simulink model "laba4"  (R2016b)
settings: Solver=VariableStepAuto  StartTime=0.0  StopTime=0.35  MaxStep=0.001  RelTol=1e-3
settings Model: Creator=Admin  LastModifiedBy=Admin

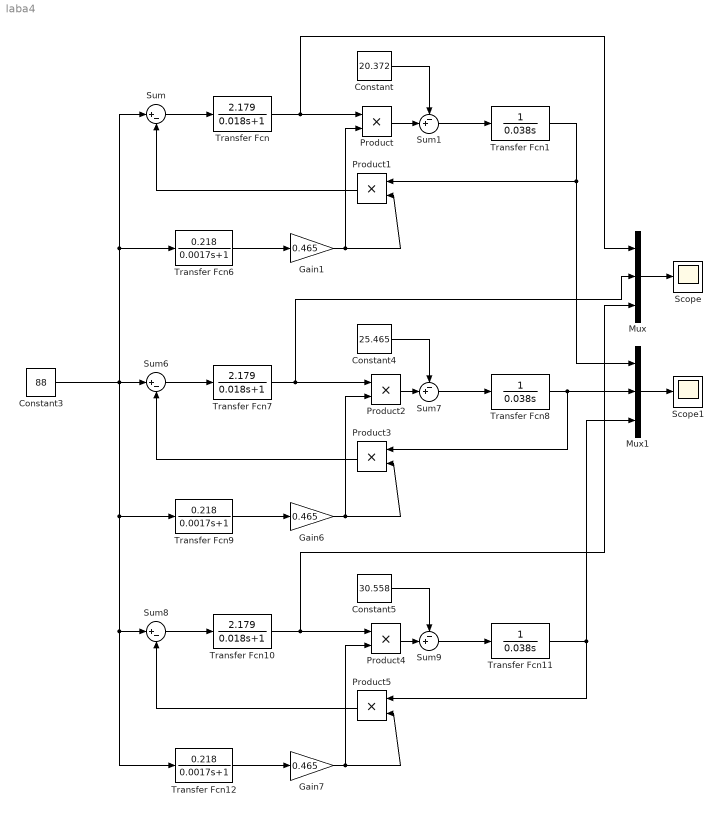
== system laba4 ==
  Constant : Constant  Value=20.372
  Constant3 : Constant  Value=88
  Constant4 : Constant  Value=25.465
  Constant5 : Constant  Value=30.558
  Gain1 : Gain  Gain=0.465
  Gain6 : Gain  Gain=0.465
  Gain7 : Gain  Gain=0.465
  Mux : Mux  Inputs=3
  Mux1 : Mux  Inputs=3
  Product{,1..5} (6 alike) : Product
  Scope : Scope
  Scope1 : Scope
  Sum : Sum  Inputs=|+-
  Sum1 : Sum  Inputs=-+|
  Sum6 : Sum  Inputs=|+-
  Sum7 : Sum  Inputs=-+|
  Sum8 : Sum  Inputs=|+-
  Sum9 : Sum  Inputs=-+|
  Transfer Fcn : TransferFcn  Numerator=[2.179]  Denominator=[0.018 1]
  Transfer Fcn1 : TransferFcn  Denominator=[0.038 0]
  Transfer Fcn10 : TransferFcn  Numerator=[2.179]  Denominator=[0.018 1]
  Transfer Fcn11 : TransferFcn  Denominator=[0.038 0]
  Transfer Fcn12 : TransferFcn  Numerator=[0.218]  Denominator=[0.0017 1]
  Transfer Fcn6 : TransferFcn  Numerator=[0.218]  Denominator=[0.0017 1]
  Transfer Fcn7 : TransferFcn  Numerator=[2.179]  Denominator=[0.018 1]
  Transfer Fcn8 : TransferFcn  Denominator=[0.038 0]
  Transfer Fcn9 : TransferFcn  Numerator=[0.218]  Denominator=[0.0017 1]
  wires:
  Sum1/1 -> Transfer Fcn1/1
  Constant/1 -> Sum1/1
  Product/1 -> Sum1/2
  Sum/1 -> Transfer Fcn/1
  Product1/1 -> Sum/2
  Mux/1 -> Scope/1
  Mux1/1 -> Scope1/1
  Transfer Fcn6/1 -> Gain1/1
  Gain1/1 -> Product/2, Product1/2
  Sum7/1 -> Transfer Fcn8/1
  Constant4/1 -> Sum7/1
  Product2/1 -> Sum7/2
  Sum6/1 -> Transfer Fcn7/1
  Transfer Fcn8/1 -> Mux1/2, Product3/1
  Product3/1 -> Sum6/2
  Transfer Fcn9/1 -> Gain6/1
  Gain6/1 -> Product2/2, Product3/2
  Sum9/1 -> Transfer Fcn11/1
  Constant5/1 -> Sum9/1
  Product4/1 -> Sum9/2
  Transfer Fcn10/1 -> Mux/3, Product4/1
  Sum8/1 -> Transfer Fcn10/1
  Product5/1 -> Sum8/2
  Constant3/1 -> Transfer Fcn9/1, Sum8/1, Transfer Fcn12/1, Sum/1, Transfer Fcn6/1, Sum6/1
  Transfer Fcn12/1 -> Gain7/1
  Gain7/1 -> Product4/2, Product5/2
  Transfer Fcn/1 -> Mux/1, Product/1
  Transfer Fcn7/1 -> Mux/2, Product2/1
  Transfer Fcn1/1 -> Product1/1, Mux1/1
  Transfer Fcn11/1 -> Product5/1, Mux1/3
